simulink model "mod_massa_molla"  (Simulink 7.6)
settings: Solver=ode45  StartTime=0.0  StopTime=10.0  MaxStep=.01  RelTol=1e-3
values from neighbouring files (symbols this model uses):
  A = [0 1;-k/m -b/m]    [massamollasmorz.m]    (also in serbatoi.m = [ -k1/S1 0; k1/S2 -k2/S2 ])
  B = [0;1/m]    [massamollasmorz.m]    (also in serbatoi.m = [ 1/S1; 0 ])
  C = [1 0]    [massamollasmorz.m]    (also in serbatoi.m = [0 k2])
  D = 0    [massamollasmorz.m]    (also in serbatoi.m)
  ueq = 2    [massamollasmorz.m]    (also in serbatoi.m = 1)
  x0 = [0 0]'    [massamollasmorz.m]    (also in serbatoi.m = [1 1]')
libraries: simulink x1
settings Model: Creator=patrizio  LastModifiedBy=patrizio

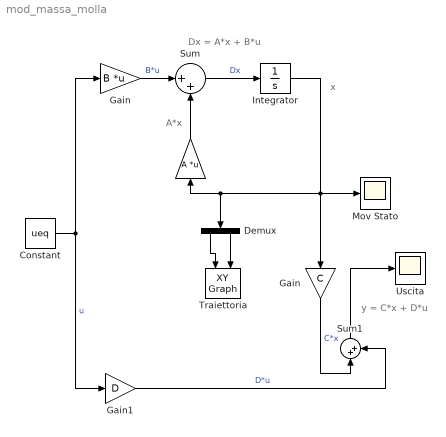
== system mod_massa_molla ==
  note: A*x
  note: Dx = A*x + B*u
  note: y = C*x + D*u
  note: x
  " " : Gain  Gain=A  Multiplication=Matrix(K*u)
  " Gain" : Gain  Gain=B  Multiplication=Matrix(K*u)
  Constant : Constant  Value=ueq
  Demux : Demux  Outputs=2
  Gain : Gain  Gain=C
  Gain1 : Gain  Gain=D
  Integrator : Integrator  InitialCondition=x0
  Mov Stato : Scope
      settings: TimeRange=10  YMin=0  YMax=8
  Sum : Sum  Inputs=|++
  Sum1 : Sum  Inputs=|++
  Traiettoria : simulink/Sinks/XY Graph  SystemSampleTime=-1  xmin=0  xmax=8  ymin=0  ymax=2  st=-1
  Uscita : Scope
  wires:
  " Gain"/1 -> Sum/1  "B*u"
  " "/1 -> Sum/2
  Constant/1 -> " Gain"/1, Gain1/1  "u"
  Integrator/1 -> Gain/1, Mov Stato/1, " "/1, Demux/1
  Sum/1 -> Integrator/1  "Dx"
  Gain/1 -> Sum1/1  "C*x"
  Gain1/1 -> Sum1/2  "D*u"
  Sum1/1 -> Uscita/1
  Demux/2 -> Traiettoria/2
  Demux/1 -> Traiettoria/1
